simulink model "Compare_IcestorageWP2Measurement"  (R2018b)
settings: Solver=ode45  StartTime=0  StopTime=(31+29+31+30+31+30+31+14)*24*3600  RelTol=1e-3  EnableMultiTasking=on
undefined symbols (not defined in the file or in its folder): path_carnot
libraries: carnot x39, simulink x4
(part 1 of 2)
settings Model: SimulationMode=accelerator  Creator=U_13.adm_zivi  LastModifiedBy=drhf
settings DataIOCC: SaveFormat=Array  SignalLoggingSaveFormat=ModelDataLogs  SaveOutput=off  SignalLogging=off  SaveTime=off
settings OptimizationCC: ExpressionDepthLimit=2147483647  LifeSpan=inf
settings DebuggingCC: UnderspecifiedInitializationDetection=Classic  MergeDetectMultiDrivingBlocksExec=none  SolverPrmCheckMsg=warning  FcnCallInpInsideContextMsg=warning  StateNameClashWarn=warning  SFUnexpectedBacktrackingDiag=warning  SFNoUnconditionalDefaultTransitionDiag=warning  SFExecutionAtInitializationDiag=none
settings HardwareCC: ProdBitPerPointer=32  ProdBitPerSizeT=32  ProdBitPerPtrDiffT=32  ProdLargestAtomicFloat=None  ProdIntDivRoundTo=Undefined  ProdEndianess=Unspecified  ProdWordSize=32  ProdHWDeviceType=32-bit Generic
settings ModelReferenceCC: PropagateSignalLabelsOutOfModel=off
settings SFSimCC: SimUseLocalCustomCode=off
settings RTWCC: RTWUseLocalCustomCode=off
settings CodeAppCC: StateflowObjectComments=on
settings GRTTargetCC: TargetLangStandard=C89/C90 (ANSI)  GeneratePreprocessorConditionals=Disable all  CombineOutputUpdateFcns=off  GRTInterface=on
settings ConfigComp: CovMetricSettings=dw  CovHtmlReporting=on  CovSaveCumulativeToWorkspaceVar=on  CovSaveSingleToWorkspaceVar=on  CovExternalEMLEnable=off

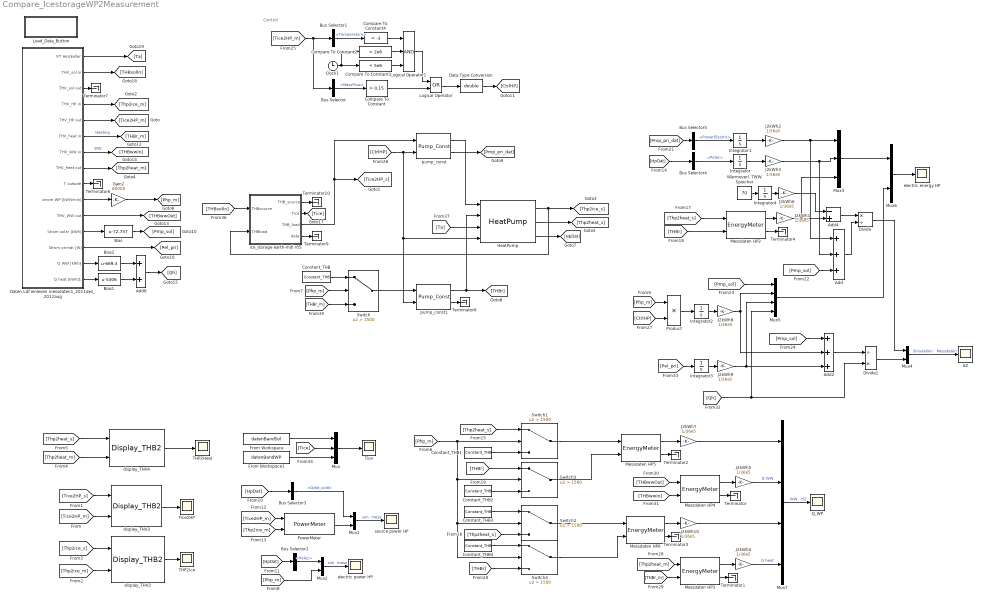
== system Compare_IcestorageWP2Measurement ==
  note: Control
  AZ : Scope
  Add : Sum  Inputs=+++
  Add2 : Sum  Inputs=+++
  Add4 : Sum  Inputs=-+
  Add8 : Sum
  Bias : Bias  Bias=-72.757
  Bias1 : Bias  Bias=-5306
  Bias2 : Bias  Bias=-669.3
  Bus Selector : BusSelector  OutputSignals=MassFlow
  Bus Selector1 : BusSelector  OutputSignals=Temperature
  Bus Selector2 : BusSelector  OutputSignals=Pelec
  Bus Selector3 : BusSelector  OutputSignals=Qdot_cold
  Bus Selector4 : BusSelector  OutputSignals=Pelec
  Bus Selector5 : BusSelector  OutputSignals=PowerElectric
  Clock1 : Clock
  Compare To Constant : simulink/Logic and Bit Operations/Compare To Constant  relop=>  const=0.15  OutDataTypeStr=uint8
  Compare To Constant2 : simulink/Logic and Bit Operations/Compare To Constant  relop=>  const=2e6  OutDataTypeStr=uint8
  Compare To Constant3 : simulink/Logic and Bit Operations/Compare To Constant  relop=<  const=5e6  OutDataTypeStr=uint8
  Compare To Constant4 : simulink/Logic and Bit Operations/Compare To Constant  relop=<  const=-3  OutDataTypeStr=uint8
  Constant_THB{,1..4} (5 alike) : carnot/Source/Simple/Constant_THB  t=20  mdot=0  p=1e5  mID=No Pressure Drop  fluid=Water  mix=0  mix2=0  mix3=0  dia=0.02  hgt=0
      settings: SourceProductName=Carnot
  Data Type Conversion : DataTypeConversion  OutDataTypeStr=double
  Daten Ldf einlesen messdaten1_2011dez_2012aug : Subsystem
  Divide : Product  Inputs=*/
  Divide1 : Product  Inputs=/*
  From Workspace : FromWorkspace  VariableName=datenBandSol  SampleTime=60
  From Workspace1 : FromWorkspace  VariableName=datenBandWP  SampleTime=60
  Gain2 : Gain  Gain=60000
  HeatPump : carnot/Source/Heat_Pump/HeatPump  PathName=fullfile(path_carnot('intlibsl'), 'Source', 'Heat_Pump', 'HeatPump', 'parameter_set')  FileName='<user defined>'  userPath=off  userParam=on  K=[172.666667120004 -31.000000610212 7095.00002905086 -6.33333383294697 42.2499995181333 -136.249984347629 178.999999113974 -70.2500000918737 7221.25000248006]  caph=25000  capc=25000  UA=5  relQdotMin=1  linc=10  quac=100  linh=10  quah=100
      settings: SourceProductName=Carnot
  Integrator{,1..4} (5 alike) : Integrator
  J2kWh{1..10} (10 alike) : Gain  Gain=1/36e5  SaturateOnIntegerOverflow=on  OutDataTypeStr=Inherit: Same as input  ParamDataTypeStr=Inherit: Same as input
  Load_Data_Button : Subsystem
      settings: OpenFcn=|
      | [filename, pathname, filterindex] = ...
      |    uigetfile( {'*.mat','MAT-files (*.mat)'; ...
      |    '*.*',  'All Files (*.*)'},  'Pick a data file');
      | 
      | if (filterindex > 0)
      |    load(filename)
      | end
      mask Display: disp('double click \nto load data')
  Logical Operator : Logic  Operator=OR  AllPortsSameDT=off  OutDataTypeStr=boolean
  Logical Operator1 : Logic  Inputs=3  AllPortsSameDT=off  OutDataTypeStr=boolean
  Messdaten HP{2..6} (5 alike) : carnot/Control/EnergyMeter
      settings: SourceProductName=Carnot
  Mux : Mux  Inputs=3
  Mux{1..2,4,6} (4 alike) : Mux  Inputs=2
  Mux3 : Mux  Inputs=3
  Mux5 : Mux
  Mux7 : Mux
  PowerMeter : carnot/Control/PowerMeter
      settings: SourceProductName=Carnot
  Product : Product  RndMeth=Zero
  Q_WP : Scope
  Switch{,1..4} (5 alike) : Switch  Criteria=u2 > Threshold  Threshold=1500
  THP2Heat : Scope
  THP2Ice : Scope
  Terminator{,1..4,6..10} (10 alike) : Terminator
  Tice : Scope
  Tice2HP : Scope
  Wärmeverl. TWW Speicher : Constant  Value=70
  display_THV2 : carnot/Outputs/Display_THB2  t=on  m=off  p=off  id=off  mix=off  d=off
      settings: SourceProductName=Carnot
  display_THV3 : carnot/Outputs/Display_THB2  t=on  m=off  p=off  id=off  mix=off  d=off
      settings: SourceProductName=Carnot
  display_THV4 : carnot/Outputs/Display_THB2  t=on  m=off  p=off  id=off  mix=off  d=off
      settings: SourceProductName=Carnot
  electric energy HP : Scope
  electric power HP : Scope
  ice_storage earth-mdl r05 : Subsystem  mask(simple water storage){vol=10, l_solar=195, l_hp=7*50, f_ice=0, t_ini=1, z=3.32-0.12, h=2.3, dearth=0.5, Tmeanoutside=11, deltathetae=9.3, Tmeaninside=5, deltathetai=15, tshift=319, cond_ground=2, cp_ground=800, rho_ground=2500}
      mask prompts: vol "volume [m³]"; l_solar "length of solar heat exchanger [m]"; l_hp "length of HP heat exchanger [m]"; f_ice "Initial fraction of ice (0..1)"; t_ini "Initial Temperatur (only if fraction ice = 0) [°C]"; z "depth of baseplate from upper surface [m]"; h "height of ice storage [m]"; dearth "thickness of surrounding earth layer [m]"; Tmeanoutside "mean outside temperature over one year [°C]"; deltathetae "amplitude of monthly outside temperatures [°C]"; Tmeaninside "mean inside temperature over one year [°C]"; deltathetai "amplitude of monthly mean inside temperature [°C]"; tshift "time shift where external temperature sine-curve shows a minimum [h]"; cond_ground "conductivity of ground [W/(m*K)]"; cp_ground "capacity of ground [J/(kg*K)]"; rho_ground "density of ground [kg/m^3]"
      mask help: multinode water storage
      mask init:
      | f_ice = min(1, max(0, f_ice));
      | h_ini = (1-f_ice)*335e3;
      | if f_ice == 0 
      |     h_ini = h_ini + 4182*t_ini;
      | end
      | %Durchmesser Eisspeicher [m]
      | D_tank = 2.7;
      | %Höhe Eisspeicher [m]
      | h_tank = 2.3;
      | %Grundfläche [m^2]
      | A = pi*(D_tank/2.)^2;
      | %Umfang [m]
      | P = D_tank*pi;
      | %charakteristisches Bodenmass [m]
      | B = A/(0.5*P);
      | %Wärmewiderstand Boden & Wand [m^2*K/W]
      | Rbtot = 0.12/1.330;
      | Rwtot = 0.1/1.330;
      | %Wanddicke [m]
      | w = 0.1;
      | %wirksame Dicke Boden & Wand [m]
      | dt = w + cond_ground*Rbtot;
      | dw = cond_ground*Rwtot;
      | %abstand der mitte der wandfläche zur oberfläche [m]
      | ztilde = z-(0.5*h);
      | %anzahl stunden pro jahr
      | t0 = 8760;
      | %thermische eindringtiefe
      | delta_grd = sqrt((t0*3600*cond_ground)/(pi*rho_ground*cp_ground));
      | 
      | %U-Wert Erdschicht [W/m^2K]
      | U_earth = cond_ground/dearth;
      | %Oberfläche Erdschicht [m^2]
      | A_earth = ((D_tank+2*dearth)/2)^2*pi + (D_tank+2*dearth)*pi*(h_tank+dearth);
      | %Volumen Erdschicht [m^3]
      | V_earth = ((D_tank+2*dearth)/2)^2*pi*(h_tank+dearth) - (D_tank/2)^2*pi*h_tank;
      | %U*A tank
      | UA_tank = (D_tank/2)^2*pi/(0.12/1.330) + D_tank*pi*h_tank/(0.1/1.330);
      mask Help: eval('man(''storage'')')
      mask Display: plot(0,0,100,100,[20,30,40,50,60,70,70,60,50,40,30,20,20],[70,90,84,84,90,70,20,13,10,10,13,20,70],[60,50,40,30],[90,95,95,90],[70,60,50,40,30,20],[70,64,60,60,64,70],[45,45],[20,50],[56,35],[35,35],[53,37],[26,44],[53,37],[44,26],[48,45,42],[46,43,46],[54,51,54],[33,35,38],[48,45,42],[24,28,23],[37,40,37],[32,35,38])
  pump_const : carnot/Hydraulics/Pump_Const  mdotmax=0.2  dia=0.0157  p0=1e5  fluid_id=Water  mix=0.5  mix2=0  mix3=0  UA=0  mcp=4182  Tini=20  e0=10  e1=10  e2=-1
      settings: SourceProductName=Carnot
  pump_const1 : carnot/Hydraulics/Pump_Const  mdotmax=0.52  dia=0.0157  p0=3e5  fluid_id=Water  mix=0  mix2=0  mix3=0  UA=0  mcp=4182  Tini=20  e0=10  e1=10  e2=-1
      settings: SourceProductName=Carnot
  source power HP : Scope
  wires:
  HeatPump/1 -> [Thp2ice_s], ice_storage earth-mdl r05/2(THBload)
  ice_storage earth-mdl r05/3(THB_load) -> pump_const/1, [Tice2HP_s]
  pump_const/1 -> HeatPump/1
  [Ta] -> HeatPump/3
  [THBsolIn] -> ice_storage earth-mdl r05/1(THBsource)
  Daten Ldf einlesen messdaten1_2011dez_2012aug/5(THV_HP out) -> [Tice2HP_m]
  [CtrlHP] -> HeatPump/4, pump_const1/2, pump_const/2
  Mux/1 -> Tice/1
  From Workspace/1 -> Mux/1
  From Workspace1/1 -> Mux/3
  display_THV2/1 -> THP2Ice/1
  Daten Ldf einlesen messdaten1_2011dez_2012aug/6(THV_heat in) -> [THBr_m]  "Heating"
  pump_const1/1 -> [THBr], HeatPump/2
  display_THV4/1 -> THP2Heat/1
  Daten Ldf einlesen messdaten1_2011dez_2012aug/7(THV_WW in) -> [THBwwIn]  "WW"
  [Tice] -> Mux/2
  [HpDat] -> Bus Selector3/1
  Daten Ldf einlesen messdaten1_2011dez_2012aug/4(THV_HP in) -> [Thp2ice_m]
  Mux1/1 -> source power HP/1  "sim  mess"
  display_THV3/1 -> Tice2HP/1
  Daten Ldf einlesen messdaten1_2011dez_2012aug/10(strom WP [kWH/min]) -> Gain2/1
  Bus Selector3/1 -> Mux1/1  "<Qdot_cold>"
  PowerMeter/1 -> Mux1/2
  Bus Selector2/1 -> Mux2/1  "<Pelec>"
  Mux2/1 -> electric power HP/1  "sim  mess"
  HeatPump/2 -> [Thp2heat_s]
  Compare To Constant/1 -> Logical Operator/2
  Logical Operator/1 -> Data Type Conversion/1
  Switch/1 -> pump_const1/1
  Constant_THB/1 -> Switch/1
  Daten Ldf einlesen messdaten1_2011dez_2012aug/8(THV_heat out) -> [Thp2heat_m]
  Clock1/1 -> Compare To Constant3/1, Compare To Constant2/1
  Compare To Constant2/1 -> Logical Operator1/2
  Compare To Constant3/1 -> Logical Operator1/3
  Bus Selector1/1 -> Compare To Constant4/1  "<Temperature>"
  Compare To Constant4/1 -> Logical Operator1/1
  Logical Operator1/1 -> Logical Operator/1
  Messdaten HP2/1 -> J2kWh1/1
  [Pmp_pri_dat] -> Bus Selector5/1
  Integrator1/1 -> J2kWh2/1
  Integrator/1 -> J2kWh3/1
  J2kWh2/1 -> Mux3/1, Add/1
  J2kWh3/1 -> Mux3/2, Add/2
  J2kWh1/1 -> Mux3/3, Add4/2
  Add/1 -> Divide/2
  Bus Selector/1 -> Compare To Constant/1  "<MassFlow>"
  [Php_m] -> Switch4/2, Switch2/2, Switch3/2, Switch1/2
  Messdaten HP3/1 -> J2kWh4/1
  Messdaten HP4/1 -> J2kWh5/1
  Daten Ldf einlesen messdaten1_2011dez_2012aug/11(THV_WW out) -> [THBwwOut]
  J2kWh4/1 -> Mux7/4  "Q heat"
  J2kWh5/1 -> Mux7/2  "Q WW"
  [Pel_pri] -> Integrator3/1
  Integrator2/1 -> J2kWh8/1
  Integrator3/1 -> J2kWh9/1
  Add2/1 -> Divide1/1
  Divide/1 -> Mux4/1
  Divide1/1 -> Mux4/2
  Mux4/1 -> AZ/1  "Simulation   Messdaten"
  Product/1 -> Integrator2/1
  Mux5/1 -> Mux6/2
  Mux3/1 -> Mux6/1
  Mux6/1 -> electric energy HP/1
  J2kWh8/1 -> Add2/2, Mux5/2
  J2kWh9/1 -> Mux5/3, Add2/3
  Daten Ldf einlesen messdaten1_2011dez_2012aug/12(Strom solar [kWh]) -> Bias/1
  Wärmeverl. TWW Speicher/1 -> Integrator4/1
  Integrator4/1 -> J2kWh6/1
  J2kWh6/1 -> Add4/1
  Add4/1 -> Divide/1
  Switch1/1 -> Messdaten HP5/1
  Switch3/1 -> Messdaten HP5/2
  Switch2/1 -> Messdaten HP6/1
  Switch4/1 -> Messdaten HP6/2
  Messdaten HP5/1 -> J2kWh7/1
  Messdaten HP6/1 -> J2kWh10/1
  J2kWh7/1 -> Mux7/1
  J2kWh10/1 -> Mux7/3
  Mux7/1 -> Q_WP/1  "WW   HZ"
  Bias2/1 -> Add8/1
  Daten Ldf einlesen messdaten1_2011dez_2012aug/14(Q WW [kWh]) -> Bias2/1
  Daten Ldf einlesen messdaten1_2011dez_2012aug/15(Q heat [kWh]1) -> Bias1/1
  [Qh] -> Divide1/2, Mux5/4
  Messdaten HP4/2 -> Terminator/1
  Messdaten HP3/2 -> Terminator1/1
  Messdaten HP5/2 -> Terminator2/1
  Messdaten HP6/2 -> Terminator3/1
  Messdaten HP2/2 -> Terminator4/1
  Daten Ldf einlesen messdaten1_2011dez_2012aug/9(T outside) -> Terminator6/1
  Daten Ldf einlesen messdaten1_2011dez_2012aug/3(THV_sol out) -> Terminator7/1
  pump_const1/2 -> Terminator8/1
  ice_storage earth-mdl r05/4(data) -> Terminator9/1
  ice_storage earth-mdl r05/1(THB_source) -> Terminator10/1
  Constant_THB1/1 -> Switch1/3
  Constant_THB2/1 -> Switch3/3
  Constant_THB3/1 -> Switch2/1
  Constant_THB4/1 -> Switch4/1
  [Tice2HP_m] -> display_THV3/2
  [Tice2HP_s] -> display_THV3/1
  [Thp2ice_m] -> display_THV2/2
  [Thp2ice_s] -> display_THV2/1
  [Thp2heat_m] -> display_THV4/2
  [Thp2heat_s] -> display_THV4/1
  Gain2/1 -> [Php_m]
  [Php_m] -> Switch/2
  [Php_m] -> Mux2/2
  [Php_m] -> Product/1
  HeatPump/3 -> [HpDat]
  [HpDat] -> Bus Selector2/1
  [Tice2HP_m] -> PowerMeter/1
  [Thp2ice_m] -> PowerMeter/2
  [HpDat] -> Bus Selector4/1
  Bus Selector4/1 -> Integrator/1  "<Pelec>"
  [Thp2heat_s] -> Switch1/1
  [Thp2heat_s] -> Switch2/3
  [Thp2heat_s] -> Messdaten HP2/1
  [THBr] -> Messdaten HP2/2
  [THBr] -> Switch3/1
  [THBr] -> Switch4/3
  pump_const/2 -> [Pmp_pri_dat]
  Bus Selector5/1 -> Integrator1/1  "<PowerElectric>"
  [Pmp_sol] -> Add/3
  [Pmp_sol] -> Mux5/1
  [Pmp_sol] -> Add2/1
  Bias/1 -> [Pmp_sol]
  Bias1/1 -> Add8/2
  [Tice2HP_m] -> Bus Selector/1, Bus Selector1/1
  Data Type Conversion/1 -> [CtrlHP]
  [CtrlHP] -> Product/2
  [Thp2heat_m] -> Messdaten HP3/1
  [THBr_m] -> Messdaten HP3/2
  [THBwwOut] -> Messdaten HP4/1
  [THBwwIn] -> Messdaten HP4/2
  Add8/1 -> [Qh]
  Daten Ldf einlesen messdaten1_2011dez_2012aug/13(Strom primär [W]) -> [Pel_pri]
  ice_storage earth-mdl r05/2(Tice) -> [Tice]
  [THBr_m] -> Switch/3
  Daten Ldf einlesen messdaten1_2011dez_2012aug/2(THV_sol in) -> [THBsolIn]
  Daten Ldf einlesen messdaten1_2011dez_2012aug/1(RT Heizkeller) -> [Ta]

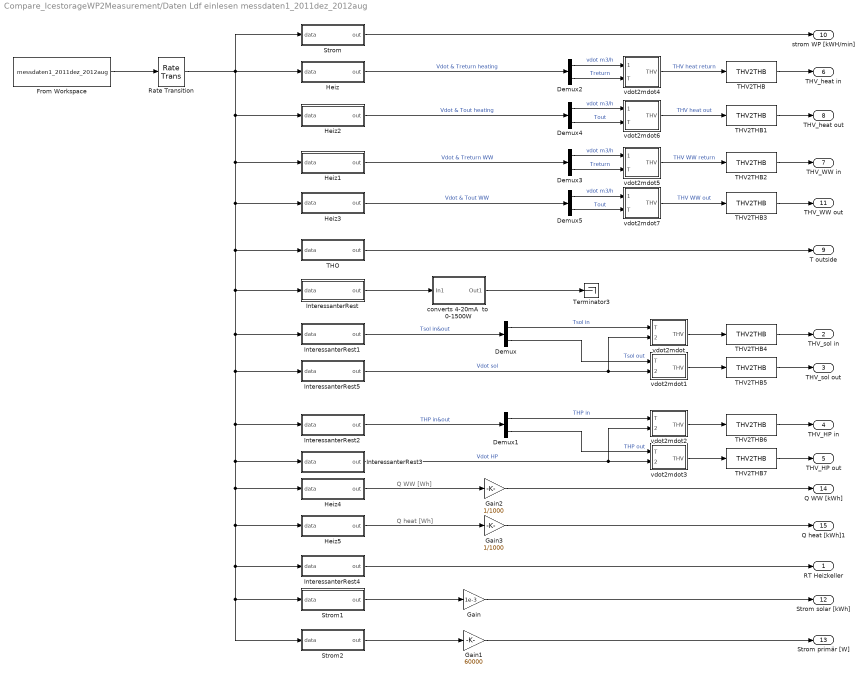
== system Compare_IcestorageWP2Measurement/Daten Ldf einlesen messdaten1_2011dez_2012aug ==
  note: Q WW [Wh]
  note: Q heat [Wh]
  Demux{,1..5} (6 alike) : Demux  Outputs=2
  From Workspace : FromWorkspace  VariableName=messdaten1_2011dez_2012aug  SampleTime=60  Interpolate=off  OutputAfterFinalValue=Holding final value
  Gain : Gain  Gain=1e-3
  Gain1 : Gain  Gain=60000
  Gain2 : Gain  Gain=1/1000
  Gain3 : Gain  Gain=1/1000
  Heiz : Subsystem  mask(Selector Messdaten Viessmann){a1=off, a2=off, a3=on, a4=off, a5=on, a6=off, a7=off, a8=off, a9=off, a10=off}
      mask prompts: a1 "Heizkreis_Wh [NONE]"; a2 "Heizkreis_m3 [NONE]"; a3 "Heizkreis_m3/h [NONE]"; a4 "Heizkreis_Tflow [NONE]"; a5 "Heizkreis_Treturn [NONE]"; a6 "TWW+Zirkulation_Wh [NONE]"; a7 "TWW+Zirkulation_m3 [NONE]"; a8 "TWW+Zirkulation_m3/h [NONE]"; a9 "TWW+Zirkulation_Tflow [NONE]"; a10 "TWW+Zirkulation_Treturn [NONE]"
      mask help:
      | Wählt die Messdaten der Viessmann Eisspeicher Anlage aus.
      | Daten der Messungen:
      | Dezember 2011 - August 2012
      mask init:
      | v=[];
      | if (a1)  v = [4];     end
      | if (a2)  v = [v 5];     end
      | if (a3)  v = [v 6];    end
      | if (a4)  v = [v 7];    end
      | if (a5)  v = [v 8];    end
      | if (a6)  v = [v 29];    end
      | if (a7)  v = [v 30];    end
      | if (a8)  v = [v 31];    end
      | if (a9)  v = [v 32];    end
      | if (a10)  v = [v 33];    end
      | if (~numel(v)) v = [6]; end
  Heiz1 : Subsystem  mask(Selector Messdaten Viessmann){a1=off, a2=off, a3=off, a4=off, a5=off, a6=off, a7=off, a8=on, a9=off, a10=on}
      mask prompts: a1 "Heizkreis_Wh [NONE]"; a2 "Heizkreis_m3 [NONE]"; a3 "Heizkreis_m3/h [NONE]"; a4 "Heizkreis_Tflow [NONE]"; a5 "Heizkreis_Treturn [NONE]"; a6 "TWW+Zirkulation_Wh [NONE]"; a7 "TWW+Zirkulation_m3 [NONE]"; a8 "TWW+Zirkulation_m3/h [NONE]"; a9 "TWW+Zirkulation_Tflow [NONE]"; a10 "TWW+Zirkulation_Treturn [NONE]"
      mask help:
      | Wählt die Messdaten der Viessmann Eisspeicher Anlage aus.
      | Daten der Messungen:
      | Dezember 2011 - August 2012
      mask init: same as Compare_IcestorageWP2Measurement/Daten Ldf einlesen messdaten1_2011dez_2012aug/Heiz
  Heiz2 : Subsystem  mask(Selector Messdaten Viessmann){a1=off, a2=off, a3=on, a4=on, a5=off, a6=off, a7=off, a8=off, a9=off, a10=off}
      mask prompts: a1 "Heizkreis_Wh [NONE]"; a2 "Heizkreis_m3 [NONE]"; a3 "Heizkreis_m3/h [NONE]"; a4 "Heizkreis_Tflow [NONE]"; a5 "Heizkreis_Treturn [NONE]"; a6 "TWW+Zirkulation_Wh [NONE]"; a7 "TWW+Zirkulation_m3 [NONE]"; a8 "TWW+Zirkulation_m3/h [NONE]"; a9 "TWW+Zirkulation_Tflow [NONE]"; a10 "TWW+Zirkulation_Treturn [NONE]"
      mask help:
      | Wählt die Messdaten der Viessmann Eisspeicher Anlage aus.
      | Daten der Messungen:
      | Dezember 2011 - August 2012
      mask init: same as Compare_IcestorageWP2Measurement/Daten Ldf einlesen messdaten1_2011dez_2012aug/Heiz
  Heiz3 : Subsystem  mask(Selector Messdaten Viessmann){a1=off, a2=off, a3=off, a4=off, a5=off, a6=off, a7=off, a8=on, a9=on, a10=off}
      mask prompts: a1 "Heizkreis_Wh [NONE]"; a2 "Heizkreis_m3 [NONE]"; a3 "Heizkreis_m3/h [NONE]"; a4 "Heizkreis_Tflow [NONE]"; a5 "Heizkreis_Treturn [NONE]"; a6 "TWW+Zirkulation_Wh [NONE]"; a7 "TWW+Zirkulation_m3 [NONE]"; a8 "TWW+Zirkulation_m3/h [NONE]"; a9 "TWW+Zirkulation_Tflow [NONE]"; a10 "TWW+Zirkulation_Treturn [NONE]"
      mask help:
      | Wählt die Messdaten der Viessmann Eisspeicher Anlage aus.
      | Daten der Messungen:
      | Dezember 2011 - August 2012
      mask init: same as Compare_IcestorageWP2Measurement/Daten Ldf einlesen messdaten1_2011dez_2012aug/Heiz
  Heiz4 : Subsystem  mask(Selector Messdaten Viessmann){a1=off, a2=off, a3=off, a4=off, a5=off, a6=on, a7=off, a8=off, a9=off, a10=off}
      mask prompts: a1 "Heizkreis_Wh [NONE]"; a2 "Heizkreis_m3 [NONE]"; a3 "Heizkreis_m3/h [NONE]"; a4 "Heizkreis_Tflow [NONE]"; a5 "Heizkreis_Treturn [NONE]"; a6 "TWW+Zirkulation_Wh [NONE]"; a7 "TWW+Zirkulation_m3 [NONE]"; a8 "TWW+Zirkulation_m3/h [NONE]"; a9 "TWW+Zirkulation_Tflow [NONE]"; a10 "TWW+Zirkulation_Treturn [NONE]"
      mask help:
      | Wählt die Messdaten der Viessmann Eisspeicher Anlage aus.
      | Daten der Messungen:
      | Dezember 2011 - August 2012
      mask init: same as Compare_IcestorageWP2Measurement/Daten Ldf einlesen messdaten1_2011dez_2012aug/Heiz
  Heiz5 : Subsystem  mask(Selector Messdaten Viessmann){a1=on, a2=off, a3=off, a4=off, a5=off, a6=off, a7=off, a8=off, a9=off, a10=off}
      mask prompts: a1 "Heizkreis_Wh [NONE]"; a2 "Heizkreis_m3 [NONE]"; a3 "Heizkreis_m3/h [NONE]"; a4 "Heizkreis_Tflow [NONE]"; a5 "Heizkreis_Treturn [NONE]"; a6 "TWW+Zirkulation_Wh [NONE]"; a7 "TWW+Zirkulation_m3 [NONE]"; a8 "TWW+Zirkulation_m3/h [NONE]"; a9 "TWW+Zirkulation_Tflow [NONE]"; a10 "TWW+Zirkulation_Treturn [NONE]"
      mask help:
      | Wählt die Messdaten der Viessmann Eisspeicher Anlage aus.
      | Daten der Messungen:
      | Dezember 2011 - August 2012
      mask init: same as Compare_IcestorageWP2Measurement/Daten Ldf einlesen messdaten1_2011dez_2012aug/Heiz
  InteressanterRest : Subsystem  mask(Selector Messdaten Viessmann){a1=on, a2=off, a3=off, a4=off, a5=off, a6=off, a7=off, a8=off, a9=off, a10=off, a11=off, a12=off, a13=off, a14=off}
      mask prompts: a1 "Einstrahlung [Ampere 4-20mA=0-1500W]"; a2 "Resol  Sol-Eis VL [Celsius]"; a3 "Resol Eis-WP [m^3]"; a4 "Resol Eis-WP RL [Celsius]"; a5 "Resol Eis-WP VL [Celsius]"; a6 "Resol Sol-Eis [m^3]"; a7 "Resol Sol-Eis RL [Celsius]"; a8 "Resol Sol-WP [m^3]"; a9 "Resol Sol-WP RL [Celsius]"; a10 "Resol Sol-WP VL [Celsius]"; a11 "RT Heizkeller [Celsius]"; a12 "Ventil R2_UmschKol [Volt]"; a13 "Ventil_R3_SolPumpe [Volt]"; a14 "Ventil_R4_UmschSpe [Volt]"
      mask help:
      | Wählt die Messdaten der Viessmann Eisspeicher Anlage aus.
      | Daten der Messungen:
      | Dezember 2011 - August 2012
      mask init:
      | v=[];
      | if (a1)  v = [3];     end
      | if (a2)  v = [v 9];     end
      | if (a3)  v = [v 10];    end
      | if (a4)  v = [v 11];    end
      | if (a5)  v = [v 12];    end
      | if (a6)  v = [v 13];    end
      | if (a7)  v = [v 14];     end
      | if (a8)  v = [v 15];     end
      | if (a9)  v = [v 16];    end
      | if (a10)  v = [v 17];    end
      | if (a11)  v = [v 18];    end
      | if (a12)  v = [v 34];    end
      | if (a13)  v = [v 35];     end
      | if (a14)  v = [v 36];     end
      | if (~numel(v)) v = [6]; end
  InteressanterRest1 : Subsystem  mask(Selector Messdaten Viessmann){a1=off, a2=on, a3=off, a4=off, a5=off, a6=off, a7=on, a8=off, a9=off, a10=off, a11=off, a12=off, a13=off, a14=off}
      mask prompts: a1 "Einstrahlung [Ampere 4-20mA=0-1500W]"; a2 "Resol  Sol-Eis VL [Celsius]"; a3 "Resol Eis-WP [m^3]"; a4 "Resol Eis-WP RL [Celsius]"; a5 "Resol Eis-WP VL [Celsius]"; a6 "Resol Sol-Eis [m^3]"; a7 "Resol Sol-Eis RL [Celsius]"; a8 "Resol Sol-WP [m^3]"; a9 "Resol Sol-WP RL [Celsius]"; a10 "Resol Sol-WP VL [Celsius]"; a11 "RT Heizkeller [Celsius]"; a12 "Ventil R2_UmschKol [Volt]"; a13 "Ventil_R3_SolPumpe [Volt]"; a14 "Ventil_R4_UmschSpe [Volt]"
      mask help:
      | Wählt die Messdaten der Viessmann Eisspeicher Anlage aus.
      | Daten der Messungen:
      | Dezember 2011 - August 2012
      mask init: same as Compare_IcestorageWP2Measurement/Daten Ldf einlesen messdaten1_2011dez_2012aug/InteressanterRest
  InteressanterRest2 : Subsystem  mask(Selector Messdaten Viessmann){a1=off, a2=off, a3=off, a4=on, a5=on, a6=off, a7=off, a8=off, a9=off, a10=off, a11=off, a12=off, a13=off, a14=off}
      mask prompts: a1 "Einstrahlung [Ampere 4-20mA=0-1500W]"; a2 "Resol  Sol-Eis VL [Celsius]"; a3 "Resol Eis-WP [m^3]"; a4 "Resol Eis-WP RL [Celsius]"; a5 "Resol Eis-WP VL [Celsius]"; a6 "Resol Sol-Eis [m^3]"; a7 "Resol Sol-Eis RL [Celsius]"; a8 "Resol Sol-WP [m^3]"; a9 "Resol Sol-WP RL [Celsius]"; a10 "Resol Sol-WP VL [Celsius]"; a11 "RT Heizkeller [Celsius]"; a12 "Ventil R2_UmschKol [Volt]"; a13 "Ventil_R3_SolPumpe [Volt]"; a14 "Ventil_R4_UmschSpe [Volt]"
      mask help:
      | Wählt die Messdaten der Viessmann Eisspeicher Anlage aus.
      | Daten der Messungen:
      | Dezember 2011 - August 2012
      mask init: same as Compare_IcestorageWP2Measurement/Daten Ldf einlesen messdaten1_2011dez_2012aug/InteressanterRest
  InteressanterRest3 : Subsystem  mask(Selector Messdaten Viessmann){a1=off, a2=off, a3=on, a4=off, a5=off, a6=off, a7=off, a8=off, a9=off, a10=off, a11=off, a12=off, a13=off, a14=off}
      mask prompts: a1 "Einstrahlung [Ampere 4-20mA=0-1500W]"; a2 "Resol  Sol-Eis VL [Celsius]"; a3 "Resol Eis-WP [m^3]"; a4 "Resol Eis-WP RL [Celsius]"; a5 "Resol Eis-WP VL [Celsius]"; a6 "Resol Sol-Eis [m^3]"; a7 "Resol Sol-Eis RL [Celsius]"; a8 "Resol Sol-WP [m^3]"; a9 "Resol Sol-WP RL [Celsius]"; a10 "Resol Sol-WP VL [Celsius]"; a11 "RT Heizkeller [Celsius]"; a12 "Ventil R2_UmschKol [Volt]"; a13 "Ventil_R3_SolPumpe [Volt]"; a14 "Ventil_R4_UmschSpe [Volt]"
      mask help:
      | Wählt die Messdaten der Viessmann Eisspeicher Anlage aus.
      | Daten der Messungen:
      | Dezember 2011 - August 2012
      mask init: same as Compare_IcestorageWP2Measurement/Daten Ldf einlesen messdaten1_2011dez_2012aug/InteressanterRest
  InteressanterRest4 : Subsystem  mask(Selector Messdaten Viessmann){a1=off, a2=off, a3=off, a4=off, a5=off, a6=off, a7=off, a8=off, a9=off, a10=off, a11=on, a12=off, a13=off, a14=off}
      mask prompts: a1 "Einstrahlung [Ampere 4-20mA=0-1500W]"; a2 "Resol  Sol-Eis VL [Celsius]"; a3 "Resol Eis-WP [m^3]"; a4 "Resol Eis-WP RL [Celsius]"; a5 "Resol Eis-WP VL [Celsius]"; a6 "Resol Sol-Eis [m^3]"; a7 "Resol Sol-Eis RL [Celsius]"; a8 "Resol Sol-WP [m^3]"; a9 "Resol Sol-WP RL [Celsius]"; a10 "Resol Sol-WP VL [Celsius]"; a11 "RT Heizkeller [Celsius]"; a12 "Ventil R2_UmschKol [Volt]"; a13 "Ventil_R3_SolPumpe [Volt]"; a14 "Ventil_R4_UmschSpe [Volt]"
      mask help:
      | Wählt die Messdaten der Viessmann Eisspeicher Anlage aus.
      | Daten der Messungen:
      | Dezember 2011 - August 2012
      mask init: same as Compare_IcestorageWP2Measurement/Daten Ldf einlesen messdaten1_2011dez_2012aug/InteressanterRest
  InteressanterRest5 : Subsystem  mask(Selector Messdaten Viessmann){a1=off, a2=off, a3=off, a4=off, a5=off, a6=on, a7=off, a8=off, a9=off, a10=off, a11=off, a12=off, a13=off, a14=off}
      mask prompts: a1 "Einstrahlung [Ampere 4-20mA=0-1500W]"; a2 "Resol  Sol-Eis VL [Celsius]"; a3 "Resol Eis-WP [m^3]"; a4 "Resol Eis-WP RL [Celsius]"; a5 "Resol Eis-WP VL [Celsius]"; a6 "Resol Sol-Eis [m^3]"; a7 "Resol Sol-Eis RL [Celsius]"; a8 "Resol Sol-WP [m^3]"; a9 "Resol Sol-WP RL [Celsius]"; a10 "Resol Sol-WP VL [Celsius]"; a11 "RT Heizkeller [Celsius]"; a12 "Ventil R2_UmschKol [Volt]"; a13 "Ventil_R3_SolPumpe [Volt]"; a14 "Ventil_R4_UmschSpe [Volt]"
      mask help:
      | Wählt die Messdaten der Viessmann Eisspeicher Anlage aus.
      | Daten der Messungen:
      | Dezember 2011 - August 2012
      mask init: same as Compare_IcestorageWP2Measurement/Daten Ldf einlesen messdaten1_2011dez_2012aug/InteressanterRest
  Rate Transition : RateTransition
  Strom : Subsystem  mask(Selector Messdaten Viessmann){a1=off, a2=on, a3=off, a4=off, a5=off, a6=off}
      mask prompts: a1 "Drehstrom E-Heizst [kWh]"; a2 "Drestrom WP [kWh]"; a3 "Strom Primärpumpe [kWh]"; a4 "Strom Regelung [kWh]"; a5 "Strom Sekundärpump [kWh]"; a6 "Strom Solarstation [NONE]"
      mask help:
      | Wählt die Messdaten der Viessmann Eisspeicher Anlage aus.
      | Daten der Messungen:
      | Dezember 2011 - August 2012
      mask init:
      | v=[];
      | if (a1)  v = [1];     end
      | if (a2)  v = [v 2];     end
      | if (a3)  v = [v 19];    end
      | if (a4)  v = [v 20];    end
      | if (a5)  v = [v 21];    end
      | if (a6)  v = [v 22];    end
      | if (~numel(v)) v = [6]; end
  Strom1 : Subsystem  mask(Selector Messdaten Viessmann){a1=off, a2=off, a3=off, a4=off, a5=off, a6=on}
      mask prompts: a1 "Drehstrom E-Heizst [kWh]"; a2 "Drestrom WP [kWh]"; a3 "Strom Primärpumpe [kWh]"; a4 "Strom Regelung [kWh]"; a5 "Strom Sekundärpump [kWh]"; a6 "Strom Solarstation [NONE]"
      mask help:
      | Wählt die Messdaten der Viessmann Eisspeicher Anlage aus.
      | Daten der Messungen:
      | Dezember 2011 - August 2012
      mask init:
      | v=[];
      | if (a1)  v = [1];     end
      | if (a2)  v = [v 2];     end
      | if (a3)  v = [v 19];    end
      | if (a4)  v = [v 20];    end
      | if (a5)  v = [v 21];    end
      | if (a6)  v = [v 22];    end
      | if (~numel(v)) v = [6]; end
  Strom2 : Subsystem  mask(Selector Messdaten Viessmann){a1=off, a2=off, a3=on, a4=off, a5=off, a6=off}
      mask prompts: a1 "Drehstrom E-Heizst [kWh]"; a2 "Drestrom WP [kWh]"; a3 "Strom Primärpumpe [kWh]"; a4 "Strom Regelung [kWh]"; a5 "Strom Sekundärpump [kWh]"; a6 "Strom Solarstation [NONE]"
      mask help:
      | Wählt die Messdaten der Viessmann Eisspeicher Anlage aus.
      | Daten der Messungen:
      | Dezember 2011 - August 2012
      mask init:
      | v=[];
      | if (a1)  v = [1];     end
      | if (a2)  v = [v 2];     end
      | if (a3)  v = [v 19];    end
      | if (a4)  v = [v 20];    end
      | if (a5)  v = [v 21];    end
      | if (a6)  v = [v 22];    end
      | if (~numel(v)) v = [6]; end
  THO : Subsystem  mask(Selector Messdaten Viessmann){a1=off, a2=off, a3=off, a4=on, a5=off, a6=off}
      mask prompts: a1 "THO_rhoinst [NONE]"; a2 "THO_rhomax [NONE]"; a3 "THO_rhomin [NONE]"; a4 "THO_Tinst [NONE]"; a5 "THO_Tmax [NONE]"; a6 "THO_Tmin [NONE]"
      mask help:
      | Wählt die Messdaten der Viessmann Eisspeicher Anlage aus.
      | Daten der Messungen:
      | Dezember 2011 - August 2012
      mask init:
      | v=[];
      | if (a1)  v = [23];     end
      | if (a2)  v = [v 24];     end
      | if (a3)  v = [v 25];    end
      | if (a4)  v = [v 26];    end
      | if (a5)  v = [v 27];    end
      | if (a6)  v = [v 28];    end
      | if (~numel(v)) v = [6]; end
  THV2THB{,1..7} (8 alike) : carnot/Toolbox/THV2THB
      settings: SourceProductName=Carnot
  Terminator3 : Terminator
  converts 4-20mA  to  0-1500W : Subsystem
  vdot2mdot : Subsystem  mask(create THV){p=1e5, fluid=water_glycol_mix, mix=0.5, dia=0.025}
      mask prompts: p "pressure [Pa]"; mix "fluid mixture [0..1]"; dia "diameter [m]"
      mask help: Block to create a THV vector with the variable input T and mdot. The other value can be set as constants in the mask.
      mask init:
      | mix = min(1, max(0, mix));
      | dia = max(dia, 0.001);
      mask Help: eval('man (''create_THV'')')
      mask TypeOptions fluid: water | air | cotton_oil | silicone_oil | water_glycol_mix
  vdot2mdot1 : Subsystem  mask(create THV){p=1e5, fluid=water_glycol_mix, mix=0.5, dia=0.025}
      mask prompts: p "pressure [Pa]"; mix "fluid mixture [0..1]"; dia "diameter [m]"
      mask help: Block to create a THV vector with the variable input T and mdot. The other value can be set as constants in the mask.
      mask init:
      | mix = min(1, max(0, mix));
      | dia = max(dia, 0.001);
      mask Help: eval('man (''create_THV'')')
      mask TypeOptions fluid: water | air | cotton_oil | silicone_oil | water_glycol_mix
  vdot2mdot2 : Subsystem  mask(create THV){p=1e5, fluid=water_glycol_mix, mix=0.5, dia=0.025}
      mask prompts: p "pressure [Pa]"; mix "fluid mixture [0..1]"; dia "diameter [m]"
      mask help: Block to create a THV vector with the variable input T and mdot. The other value can be set as constants in the mask.
      mask init:
      | mix = min(1, max(0, mix));
      | dia = max(dia, 0.001);
      mask Help: eval('man (''create_THV'')')
      mask TypeOptions fluid: water | air | cotton_oil | silicone_oil | water_glycol_mix
  vdot2mdot3 : Subsystem  mask(create THV){p=1e5, fluid=water_glycol_mix, mix=0.5, dia=0.025}
      mask prompts: p "pressure [Pa]"; mix "fluid mixture [0..1]"; dia "diameter [m]"
      mask help: Block to create a THV vector with the variable input T and mdot. The other value can be set as constants in the mask.
      mask init:
      | mix = min(1, max(0, mix));
      | dia = max(dia, 0.001);
      mask Help: eval('man (''create_THV'')')
      mask TypeOptions fluid: water | air | cotton_oil | silicone_oil | water_glycol_mix
  vdot2mdot4 : Subsystem  mask(create THV){p=1e5, fluid=water, mix=0, dia=0.025}
      mask prompts: p "pressure [Pa]"; mix "fluid mixture [0..1]"; dia "diameter [m]"
      mask help: Block to create a THV vector with the variable input T and mdot. The other value can be set as constants in the mask.
      mask init:
      | mix = min(1, max(0, mix));
      | dia = max(dia, 0.001);
      mask Help: eval('man (''create_THV'')')
      mask TypeOptions fluid: water | air | cotton_oil | silicone_oil | water_glycol_mix
  vdot2mdot5 : Subsystem  mask(create THV){p=1e5, fluid=water, mix=0, dia=0.025}
      mask prompts: p "pressure [Pa]"; mix "fluid mixture [0..1]"; dia "diameter [m]"
      mask help: Block to create a THV vector with the variable input T and mdot. The other value can be set as constants in the mask.
      mask init:
      | mix = min(1, max(0, mix));
      | dia = max(dia, 0.001);
      mask Help: eval('man (''create_THV'')')
      mask TypeOptions fluid: water | air | cotton_oil | silicone_oil | water_glycol_mix
  vdot2mdot6 : Subsystem  mask(create THV){p=1e5, fluid=water, mix=0, dia=0.025}
      mask prompts: p "pressure [Pa]"; mix "fluid mixture [0..1]"; dia "diameter [m]"
      mask help: Block to create a THV vector with the variable input T and mdot. The other value can be set as constants in the mask.
      mask init:
      | mix = min(1, max(0, mix));
      | dia = max(dia, 0.001);
      mask Help: eval('man (''create_THV'')')
      mask TypeOptions fluid: water | air | cotton_oil | silicone_oil | water_glycol_mix
  vdot2mdot7 : Subsystem  mask(create THV){p=1e5, fluid=water, mix=0, dia=0.025}
      mask prompts: p "pressure [Pa]"; mix "fluid mixture [0..1]"; dia "diameter [m]"
      mask help: Block to create a THV vector with the variable input T and mdot. The other value can be set as constants in the mask.
      mask init:
      | mix = min(1, max(0, mix));
      | dia = max(dia, 0.001);
      mask Help: eval('man (''create_THV'')')
      mask TypeOptions fluid: water | air | cotton_oil | silicone_oil | water_glycol_mix
  RT Heizkeller : Outport
  THV_sol in : Outport  Port=2
  THV_sol out : Outport  Port=3
  THV_HP in : Outport  Port=4
  THV_HP out : Outport  Port=5
  THV_heat in : Outport  Port=6
  THV_WW in : Outport  Port=7
  THV_heat out : Outport  Port=8
  T outside : Outport  Port=9
  strom WP [kWH/min] : Outport  Port=10
  THV_WW out : Outport  Port=11
  Strom solar [kWh] : Outport  Port=12
  Strom primär [W] : Outport  Port=13
  Q WW [kWh] : Outport  Port=14
  Q heat [kWh]1 : Outport  Port=15
  wires:
  THO/1(out) -> T outside/1
  Heiz/1(out) -> Demux2/1  "Vdot & Treturn heating"
  converts 4-20mA  to  0-1500W/1(Out1) -> Terminator3/1
  InteressanterRest/1(out) -> converts 4-20mA  to  0-1500W/1(In1)
  Strom/1(out) -> strom WP [kWH/min]/1
  From Workspace/1 -> Rate Transition/1
  InteressanterRest1/1(out) -> Demux/1  "Tsol in&out"
  InteressanterRest2/1(out) -> Demux1/1  "THP in&out"
  InteressanterRest3/1(out) -> vdot2mdot3/2(vdot), vdot2mdot2/2(vdot)  "Vdot HP"
  InteressanterRest4/1(out) -> RT Heizkeller/1
  InteressanterRest5/1(out) -> vdot2mdot1/2(vdot), vdot2mdot/2(vdot)  "Vdot sol"
  Demux/1 -> vdot2mdot/1(T)  "Tsol in"
  Demux/2 -> vdot2mdot1/1(T)  "Tsol out"
  vdot2mdot/1(THV) -> THV2THB4/1
  vdot2mdot1/1(THV) -> THV2THB5/1
  Demux1/1 -> vdot2mdot2/1(T)  "THP in"
  Demux1/2 -> vdot2mdot3/1(T)  "THP out"
  vdot2mdot2/1(THV) -> THV2THB6/1
  vdot2mdot3/1(THV) -> THV2THB7/1
  Demux2/1 -> vdot2mdot4/1(vdot)  "vdot m3/h"
  Demux2/2 -> vdot2mdot4/2(T)  "Treturn"
  vdot2mdot4/1(THV) -> THV2THB/1  "THV heat return"
  Heiz1/1(out) -> Demux3/1  "Vdot & Treturn WW"
  Demux3/1 -> vdot2mdot5/1(vdot)  "vdot m3/h"
  Demux3/2 -> vdot2mdot5/2(T)  "Treturn"
  vdot2mdot5/1(THV) -> THV2THB2/1  "THV WW return"
  Heiz2/1(out) -> Demux4/1  "Vdot & Tout heating"
  Demux4/1 -> vdot2mdot6/1(vdot)  "vdot m3/h"
  Demux4/2 -> vdot2mdot6/2(T)  "Tout"
  vdot2mdot6/1(THV) -> THV2THB1/1  "THV heat out"
  Heiz3/1(out) -> Demux5/1  "Vdot & Tout WW"
  Demux5/1 -> vdot2mdot7/1(vdot)  "vdot m3/h"
  Demux5/2 -> vdot2mdot7/2(T)  "Tout"
  vdot2mdot7/1(THV) -> THV2THB3/1  "THV WW out"
  Strom1/1(out) -> Gain/1
  Gain/1 -> Strom solar [kWh]/1
  Strom2/1(out) -> Gain1/1
  Gain1/1 -> Strom primär [W]/1
  Heiz4/1(out) -> Gain2/1
  Gain2/1 -> Q WW [kWh]/1
  Heiz5/1(out) -> Gain3/1
  Gain3/1 -> Q heat [kWh]1/1
  THV2THB/1 -> THV_heat in/1
  THV2THB1/1 -> THV_heat out/1
  THV2THB2/1 -> THV_WW in/1
  THV2THB3/1 -> THV_WW out/1
  THV2THB4/1 -> THV_sol in/1
  THV2THB5/1 -> THV_sol out/1
  THV2THB6/1 -> THV_HP in/1
  THV2THB7/1 -> THV_HP out/1
  Rate Transition/1 -> Heiz1/1(data), InteressanterRest1/1(data), InteressanterRest2/1(data), InteressanterRest3/1(data), Heiz4/1(data), InteressanterRest4/1(data), Strom1/1(data), Strom2/1(data), Heiz5/1(data), InteressanterRest5/1(data), InteressanterRest/1(data), THO/1(data), Heiz3/1(data), Heiz2/1(data), Strom/1(data), Heiz/1(data)

== system Compare_IcestorageWP2Measurement/Load_Data_Button ==

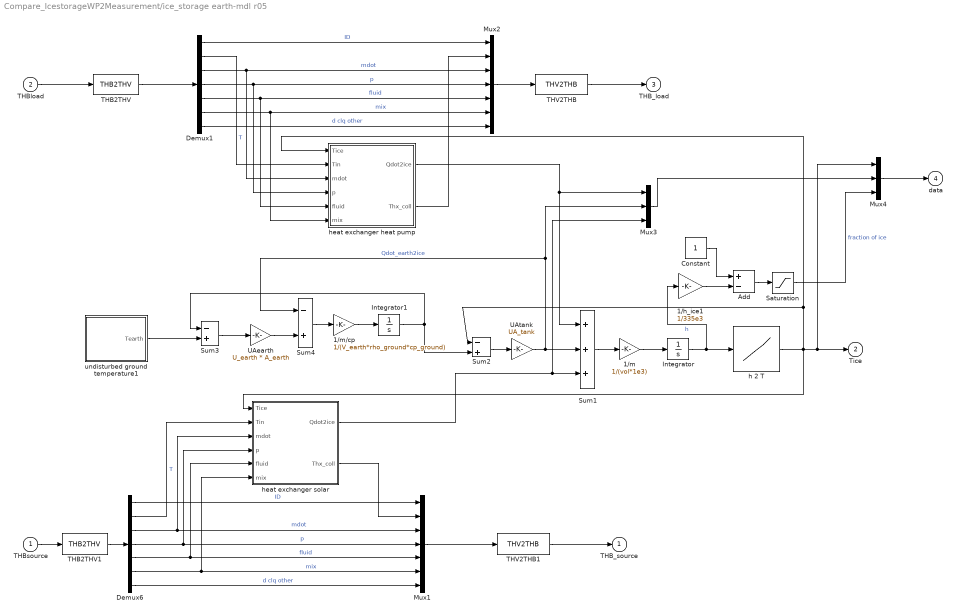
== system Compare_IcestorageWP2Measurement/ice_storage earth-mdl r05 ==
  THBsource : Inport
  THBload : Inport  Port=2
  1/h_ice1 : Gain  Gain=1/335e3  SaturateOnIntegerOverflow=on  OutDataTypeStr=Inherit: Same as input  ParamDataTypeStr=Inherit: Same as input
  1/m : Gain  Gain=1/(vol*1e3)  SaturateOnIntegerOverflow=on  OutDataTypeStr=Inherit: Same as input  ParamDataTypeStr=Inherit: Same as input
  1/m/cp : Gain  Gain=1/(V_earth*rho_ground*cp_ground)  SaturateOnIntegerOverflow=on  OutDataTypeStr=Inherit: Same as input  ParamDataTypeStr=Inherit: Same as input
  Add : Sum  Inputs=+-
  Constant : Constant
  Demux1 : Demux  Outputs=[1 1 1 1 1 1 14]
  Demux6 : Demux  Outputs=[1 1 1 1 1 1 14]
  Integrator : Integrator  InitialCondition=h_ini
  Integrator1 : Integrator  InitialCondition=4
  Mux1 : Mux  Inputs=7
  Mux2 : Mux  Inputs=7
  Mux3 : Mux  Inputs=3
  Mux4 : Mux  Inputs=3
  Saturation : Saturate  UpperLimit=1  LowerLimit=0  LinearizeAsGain=off
  Sum1 : Sum  Inputs=+++  SaturateOnIntegerOverflow=on  InputSameDT=on  OutDataTypeStr=Inherit: Same as first input
  Sum2 : Sum  Inputs=-+  SaturateOnIntegerOverflow=on  InputSameDT=on  OutDataTypeStr=Inherit: Same as first input
  Sum3 : Sum  Inputs=-+  SaturateOnIntegerOverflow=on  InputSameDT=on  OutDataTypeStr=Inherit: Same as first input
  Sum4 : Sum  Inputs=-+  SaturateOnIntegerOverflow=on  InputSameDT=on  OutDataTypeStr=Inherit: Same as first input
  THB2THV : carnot/Toolbox/THB2THV
      settings: SourceProductName=Carnot
  THB2THV1 : carnot/Toolbox/THB2THV
      settings: SourceProductName=Carnot
  THV2THB : carnot/Toolbox/THV2THB
      settings: SourceProductName=Carnot
  THV2THB1 : carnot/Toolbox/THV2THB
      settings: SourceProductName=Carnot
  UAearth : Gain  Gain=U_earth * A_earth  SaturateOnIntegerOverflow=on  OutDataTypeStr=Inherit: Same as input  ParamDataTypeStr=Inherit: Same as input
  UAtank : Gain  Gain=UA_tank  SaturateOnIntegerOverflow=on  OutDataTypeStr=Inherit: Same as input  ParamDataTypeStr=Inherit: Same as input
  h 2 T : Lookup  InputValues=[-2060*10 -2060*4 335e3 335e3+4182*10]  Table=[-10 -4 0 10]
  heat exchanger heat pump : Subsystem
  heat exchanger solar : Subsystem
  undisturbed ground temperature1 : Subsystem
  THB_source : Outport  InitialOutput=0
  Tice : Outport  Port=2  InitialOutput=0
  THB_load : Outport  Port=3  InitialOutput=0
  data : Outport  Port=4  InitialOutput=0
  wires:
  Mux3/1 -> Mux4/2
  heat exchanger heat pump/1(Qdot2ice) -> Mux3/1, Sum1/1
  heat exchanger heat pump/2(Thx_coll) -> Mux2/2
  Demux1/2 -> heat exchanger heat pump/2(Tin)  "T"
  Demux1/6 -> Mux2/6, heat exchanger heat pump/6(mix)  "mix"
  Demux1/1 -> Mux2/1  "ID"
  Demux1/7 -> Mux2/7  "d clq other"
  Demux1/5 -> Mux2/5, heat exchanger heat pump/5(fluid)  "fluid"
  Demux1/4 -> Mux2/4, heat exchanger heat pump/4(p)  "p"
  Demux1/3 -> Mux2/3, heat exchanger heat pump/3(mdot)  "mdot"
  Mux2/1 -> THV2THB/1
  THBload/1 -> THB2THV/1
  heat exchanger solar/1(Qdot2ice) -> Sum1/3, Mux3/3
  h 2 T/1 -> Sum2/1, heat exchanger heat pump/1(Tice), heat exchanger solar/1(Tice), Mux4/1, Tice/1
  Integrator1/1 -> Sum3/1, Sum2/2
  1/m/cp/1 -> Integrator1/1
  Sum4/1 -> 1/m/cp/1
  UAearth/1 -> Sum4/2
  Sum3/1 -> UAearth/1
  Integrator/1 -> h 2 T/1, 1/h_ice1/1  "h"
  UAtank/1 -> Mux3/2, Sum4/1, Sum1/2  "Qdot_earth2ice"
  Sum2/1 -> UAtank/1
  Sum1/1 -> 1/m/1
  1/m/1 -> Integrator/1
  heat exchanger solar/2(Thx_coll) -> Mux1/2
  Demux6/2 -> heat exchanger solar/2(Tin)  "T"
  Demux6/6 -> heat exchanger solar/6(mix), Mux1/6  "mix"
  Demux6/1 -> Mux1/1  "ID"
  Demux6/7 -> Mux1/7  "d clq other"
  Demux6/5 -> heat exchanger solar/5(fluid), Mux1/5  "fluid"
  Demux6/4 -> heat exchanger solar/4(p), Mux1/4  "p"
  Demux6/3 -> heat exchanger solar/3(mdot), Mux1/3  "mdot"
  Mux1/1 -> THV2THB1/1
  THBsource/1 -> THB2THV1/1
  Mux4/1 -> data/1
  1/h_ice1/1 -> Add/2
  Add/1 -> Saturation/1
  Constant/1 -> Add/1
  Saturation/1 -> Mux4/3  "fraction of ice"
  undisturbed ground temperature1/1(Tearth) -> Sum3/2
  THV2THB/1 -> THB_load/1
  THB2THV/1 -> Demux1/1
  THB2THV1/1 -> Demux6/1
  THV2THB1/1 -> THB_source/1

== system Compare_IcestorageWP2Measurement/Daten Ldf einlesen messdaten1_2011dez_2012aug/Heiz ==
  data : Inport
  Selector : Selector  InputPortWidth=36  IndexOptions=Index vector (dialog)  Indices=[v]  OutputSizes=1
  out : Outport  InitialOutput=0
  wires:
  data/1 -> Selector/1
  Selector/1 -> out/1

== system Compare_IcestorageWP2Measurement/Daten Ldf einlesen messdaten1_2011dez_2012aug/Heiz1 ==
  data : Inport
  Selector : Selector  InputPortWidth=36  IndexOptions=Index vector (dialog)  Indices=[v]  OutputSizes=1
  out : Outport  InitialOutput=0
  wires:
  Selector/1 -> out/1
  data/1 -> Selector/1

== system Compare_IcestorageWP2Measurement/Daten Ldf einlesen messdaten1_2011dez_2012aug/Heiz2 ==
  data : Inport
  Selector : Selector  InputPortWidth=36  IndexOptions=Index vector (dialog)  Indices=[v]  OutputSizes=1
  out : Outport  InitialOutput=0
  wires:
  Selector/1 -> out/1
  data/1 -> Selector/1

== system Compare_IcestorageWP2Measurement/Daten Ldf einlesen messdaten1_2011dez_2012aug/Heiz3 ==
  data : Inport
  Selector : Selector  InputPortWidth=36  IndexOptions=Index vector (dialog)  Indices=[v]  OutputSizes=1
  out : Outport  InitialOutput=0
  wires:
  data/1 -> Selector/1
  Selector/1 -> out/1

== system Compare_IcestorageWP2Measurement/Daten Ldf einlesen messdaten1_2011dez_2012aug/Heiz4 ==
  data : Inport
  Selector : Selector  InputPortWidth=36  IndexOptions=Index vector (dialog)  Indices=[v]  OutputSizes=1
  out : Outport  InitialOutput=0
  wires:
  Selector/1 -> out/1
  data/1 -> Selector/1

== system Compare_IcestorageWP2Measurement/Daten Ldf einlesen messdaten1_2011dez_2012aug/Heiz5 ==
  data : Inport
  Selector : Selector  InputPortWidth=36  IndexOptions=Index vector (dialog)  Indices=[v]  OutputSizes=1
  out : Outport  InitialOutput=0
  wires:
  data/1 -> Selector/1
  Selector/1 -> out/1

== system Compare_IcestorageWP2Measurement/Daten Ldf einlesen messdaten1_2011dez_2012aug/InteressanterRest ==
  data : Inport
  Selector : Selector  InputPortWidth=36  IndexOptions=Index vector (dialog)  Indices=[v]  OutputSizes=1
  out : Outport  InitialOutput=0
  wires:
  data/1 -> Selector/1
  Selector/1 -> out/1

== system Compare_IcestorageWP2Measurement/Daten Ldf einlesen messdaten1_2011dez_2012aug/InteressanterRest1 ==
  data : Inport
  Selector : Selector  InputPortWidth=36  IndexOptions=Index vector (dialog)  Indices=[v]  OutputSizes=1
  out : Outport  InitialOutput=0
  wires:
  Selector/1 -> out/1
  data/1 -> Selector/1

== system Compare_IcestorageWP2Measurement/Daten Ldf einlesen messdaten1_2011dez_2012aug/InteressanterRest2 ==
  data : Inport
  Selector : Selector  InputPortWidth=36  IndexOptions=Index vector (dialog)  Indices=[v]  OutputSizes=1
  out : Outport  InitialOutput=0
  wires:
  data/1 -> Selector/1
  Selector/1 -> out/1

== system Compare_IcestorageWP2Measurement/Daten Ldf einlesen messdaten1_2011dez_2012aug/InteressanterRest3 ==
  data : Inport
  Selector : Selector  InputPortWidth=36  IndexOptions=Index vector (dialog)  Indices=[v]  OutputSizes=1
  out : Outport  InitialOutput=0
  wires:
  Selector/1 -> out/1
  data/1 -> Selector/1

== system Compare_IcestorageWP2Measurement/Daten Ldf einlesen messdaten1_2011dez_2012aug/InteressanterRest4 ==
  data : Inport
  Selector : Selector  InputPortWidth=36  IndexOptions=Index vector (dialog)  Indices=[v]  OutputSizes=1
  out : Outport  InitialOutput=0
  wires:
  data/1 -> Selector/1
  Selector/1 -> out/1

== system Compare_IcestorageWP2Measurement/Daten Ldf einlesen messdaten1_2011dez_2012aug/InteressanterRest5 ==
  data : Inport
  Selector : Selector  InputPortWidth=36  IndexOptions=Index vector (dialog)  Indices=[v]  OutputSizes=1
  out : Outport  InitialOutput=0
  wires:
  data/1 -> Selector/1
  Selector/1 -> out/1

== system Compare_IcestorageWP2Measurement/Daten Ldf einlesen messdaten1_2011dez_2012aug/Strom ==
  data : Inport
  Selector : Selector  InputPortWidth=36  IndexOptions=Index vector (dialog)  Indices=[v]  OutputSizes=1
  out : Outport  InitialOutput=0
  wires:
  Selector/1 -> out/1
  data/1 -> Selector/1

== system Compare_IcestorageWP2Measurement/Daten Ldf einlesen messdaten1_2011dez_2012aug/Strom1 ==
  data : Inport
  Selector : Selector  InputPortWidth=36  IndexOptions=Index vector (dialog)  Indices=[v]  OutputSizes=1
  out : Outport  InitialOutput=0
  wires:
  data/1 -> Selector/1
  Selector/1 -> out/1

== system Compare_IcestorageWP2Measurement/Daten Ldf einlesen messdaten1_2011dez_2012aug/Strom2 ==
  data : Inport
  Selector : Selector  InputPortWidth=36  IndexOptions=Index vector (dialog)  Indices=[v]  OutputSizes=1
  out : Outport  InitialOutput=0
  wires:
  Selector/1 -> out/1
  data/1 -> Selector/1

== system Compare_IcestorageWP2Measurement/Daten Ldf einlesen messdaten1_2011dez_2012aug/THO ==
  data : Inport
  Selector : Selector  InputPortWidth=36  IndexOptions=Index vector (dialog)  Indices=[v]  OutputSizes=1
  out : Outport  InitialOutput=0
  wires:
  Selector/1 -> out/1
  data/1 -> Selector/1

== system Compare_IcestorageWP2Measurement/Daten Ldf einlesen messdaten1_2011dez_2012aug/converts 4-20mA  to  0-1500W ==
  note: converts
      | 4-20mA  to  0-1500W
  In1 : Inport
  Bias : Bias  Bias=-0.0041
  Gain : Gain  Gain=1/0.0159*1500
  Out1 : Outport
  wires:
  Gain/1 -> Out1/1
  In1/1 -> Bias/1
  Bias/1 -> Gain/1

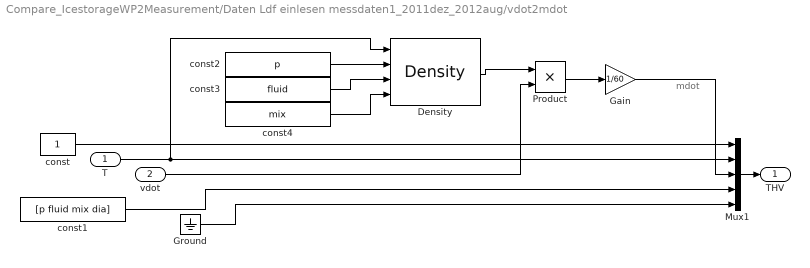
== system Compare_IcestorageWP2Measurement/Daten Ldf einlesen messdaten1_2011dez_2012aug/vdot2mdot ==
  note: mdot
  T : Inport
  vdot : Inport  Port=2
  Density : carnot/Basic/Material_Properties/Density  VariantControl=CarlibClassic  INPUTARGUMENTS=state variables (classic)  DEBUGLEVEL=DEBUGLEVEL  MAXTOTALWARNINGS=inf  MAXCONSECUTIVEWARNINGS=inf  WRITETOFILE=0  FILENAME='errors.txt'
      settings: SourceProductName=Carnot
  Gain : Gain  Gain=1/60
  Ground : Ground
  Mux1 : Mux  Inputs=[1 1 1 4 13]
  Product : Product  RndMeth=Zero
  const : Constant
  const1 : Constant  Value=[p fluid mix dia]
  const2 : Constant  Value=p
  const3 : Constant  Value=fluid
  const4 : Constant  Value=mix
  THV : Outport  InitialOutput=0
  wires:
  const1/1 -> Mux1/4
  T/1 -> Density/1, Mux1/2
  Ground/1 -> Mux1/5
  const/1 -> Mux1/1
  Mux1/1 -> THV/1
  const2/1 -> Density/2
  const3/1 -> Density/3
  const4/1 -> Density/4
  Density/1 -> Product/1
  vdot/1 -> Product/2
  Product/1 -> Gain/1
  Gain/1 -> Mux1/3

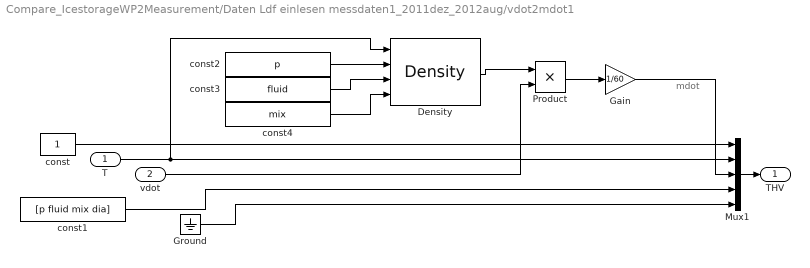
== system Compare_IcestorageWP2Measurement/Daten Ldf einlesen messdaten1_2011dez_2012aug/vdot2mdot1 ==
  note: mdot
  T : Inport
  vdot : Inport  Port=2
  Density : carnot/Basic/Material_Properties/Density  VariantControl=CarlibClassic  INPUTARGUMENTS=state variables (classic)  DEBUGLEVEL=DEBUGLEVEL  MAXTOTALWARNINGS=inf  MAXCONSECUTIVEWARNINGS=inf  WRITETOFILE=0  FILENAME='errors.txt'
      settings: SourceProductName=Carnot
  Gain : Gain  Gain=1/60
  Ground : Ground
  Mux1 : Mux  Inputs=[1 1 1 4 13]
  Product : Product  RndMeth=Zero
  const : Constant
  const1 : Constant  Value=[p fluid mix dia]
  const2 : Constant  Value=p
  const3 : Constant  Value=fluid
  const4 : Constant  Value=mix
  THV : Outport  InitialOutput=0
  wires:
  Gain/1 -> Mux1/3
  Product/1 -> Gain/1
  vdot/1 -> Product/2
  Density/1 -> Product/1
  const4/1 -> Density/4
  const3/1 -> Density/3
  const2/1 -> Density/2
  Mux1/1 -> THV/1
  const/1 -> Mux1/1
  Ground/1 -> Mux1/5
  T/1 -> Density/1, Mux1/2
  const1/1 -> Mux1/4

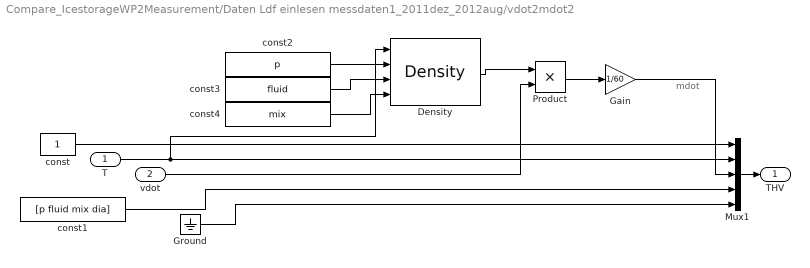
== system Compare_IcestorageWP2Measurement/Daten Ldf einlesen messdaten1_2011dez_2012aug/vdot2mdot2 ==
  note: mdot
  T : Inport
  vdot : Inport  Port=2
  Density : carnot/Basic/Material_Properties/Density  VariantControl=CarlibClassic  INPUTARGUMENTS=state variables (classic)  DEBUGLEVEL=DEBUGLEVEL  MAXTOTALWARNINGS=inf  MAXCONSECUTIVEWARNINGS=inf  WRITETOFILE=0  FILENAME='errors.txt'
      settings: SourceProductName=Carnot
  Gain : Gain  Gain=1/60
  Ground : Ground
  Mux1 : Mux  Inputs=[1 1 1 4 13]
  Product : Product  RndMeth=Zero
  const : Constant
  const1 : Constant  Value=[p fluid mix dia]
  const2 : Constant  Value=p
  const3 : Constant  Value=fluid
  const4 : Constant  Value=mix
  THV : Outport  InitialOutput=0
  wires:
  Gain/1 -> Mux1/3
  Product/1 -> Gain/1
  vdot/1 -> Product/2
  Density/1 -> Product/1
  const4/1 -> Density/4
  const3/1 -> Density/3
  const2/1 -> Density/2
  Mux1/1 -> THV/1
  const/1 -> Mux1/1
  Ground/1 -> Mux1/5
  T/1 -> Density/1, Mux1/2
  const1/1 -> Mux1/4

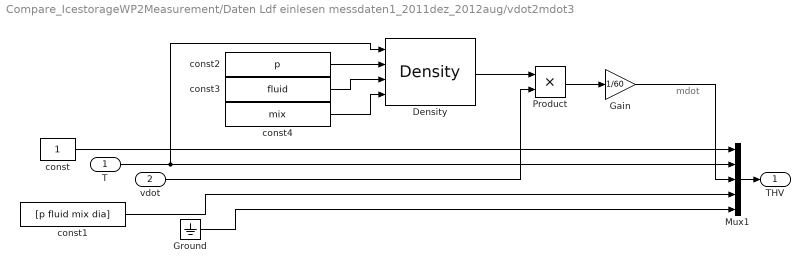
== system Compare_IcestorageWP2Measurement/Daten Ldf einlesen messdaten1_2011dez_2012aug/vdot2mdot3 ==
  note: mdot
  T : Inport
  vdot : Inport  Port=2
  Density : carnot/Basic/Material_Properties/Density  VariantControl=CarlibClassic  INPUTARGUMENTS=state variables (classic)  DEBUGLEVEL=DEBUGLEVEL  MAXTOTALWARNINGS=inf  MAXCONSECUTIVEWARNINGS=inf  WRITETOFILE=0  FILENAME='errors.txt'
      settings: SourceProductName=Carnot
  Gain : Gain  Gain=1/60
  Ground : Ground
  Mux1 : Mux  Inputs=[1 1 1 4 13]
  Product : Product  RndMeth=Zero
  const : Constant
  const1 : Constant  Value=[p fluid mix dia]
  const2 : Constant  Value=p
  const3 : Constant  Value=fluid
  const4 : Constant  Value=mix
  THV : Outport  InitialOutput=0
  wires:
  const1/1 -> Mux1/4
  T/1 -> Density/1, Mux1/2
  Ground/1 -> Mux1/5
  const/1 -> Mux1/1
  Mux1/1 -> THV/1
  const2/1 -> Density/2
  const3/1 -> Density/3
  const4/1 -> Density/4
  Density/1 -> Product/1
  vdot/1 -> Product/2
  Product/1 -> Gain/1
  Gain/1 -> Mux1/3

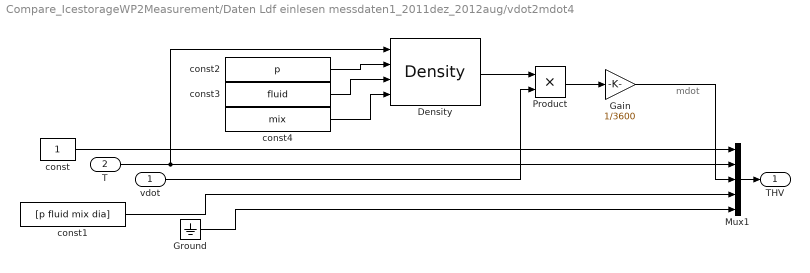
== system Compare_IcestorageWP2Measurement/Daten Ldf einlesen messdaten1_2011dez_2012aug/vdot2mdot4 ==
  note: mdot
  vdot : Inport
  T : Inport  Port=2
  Density : carnot/Basic/Material_Properties/Density  VariantControl=CarlibClassic  INPUTARGUMENTS=state variables (classic)  DEBUGLEVEL=DEBUGLEVEL  MAXTOTALWARNINGS=inf  MAXCONSECUTIVEWARNINGS=inf  WRITETOFILE=0  FILENAME='errors.txt'
      settings: SourceProductName=Carnot
  Gain : Gain  Gain=1/3600
  Ground : Ground
  Mux1 : Mux  Inputs=[1 1 1 4 13]
  Product : Product  RndMeth=Zero
  const : Constant
  const1 : Constant  Value=[p fluid mix dia]
  const2 : Constant  Value=p
  const3 : Constant  Value=fluid
  const4 : Constant  Value=mix
  THV : Outport  InitialOutput=0
  wires:
  Product/1 -> Gain/1
  vdot/1 -> Product/2
  Density/1 -> Product/1
  const4/1 -> Density/4
  const3/1 -> Density/3
  const2/1 -> Density/2
  Mux1/1 -> THV/1
  const/1 -> Mux1/1
  Ground/1 -> Mux1/5
  T/1 -> Density/1, Mux1/2
  const1/1 -> Mux1/4
  Gain/1 -> Mux1/3
